simulink model "nonlinear_simulation_stabilization"  (R2023a)
settings: Solver=VariableStepAuto  StartTime=0.0  StopTime=10.0  RelTol=1e-3
model workspace: external: MATLAB File C:\Uni\Projektarbeit\matlab\nonlinear_fo_prep.m (data not in the file)
undefined symbols (not defined in the file): C_out, init_cond
settings Model: Creator=morit  LastModifiedBy=morit

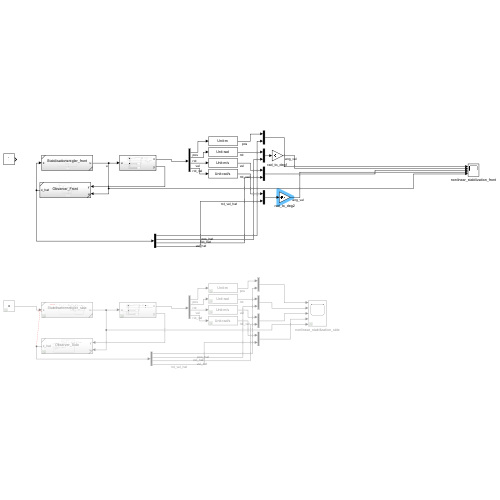
[thumbnail: Simulink's stored preview of the top-level diagram]
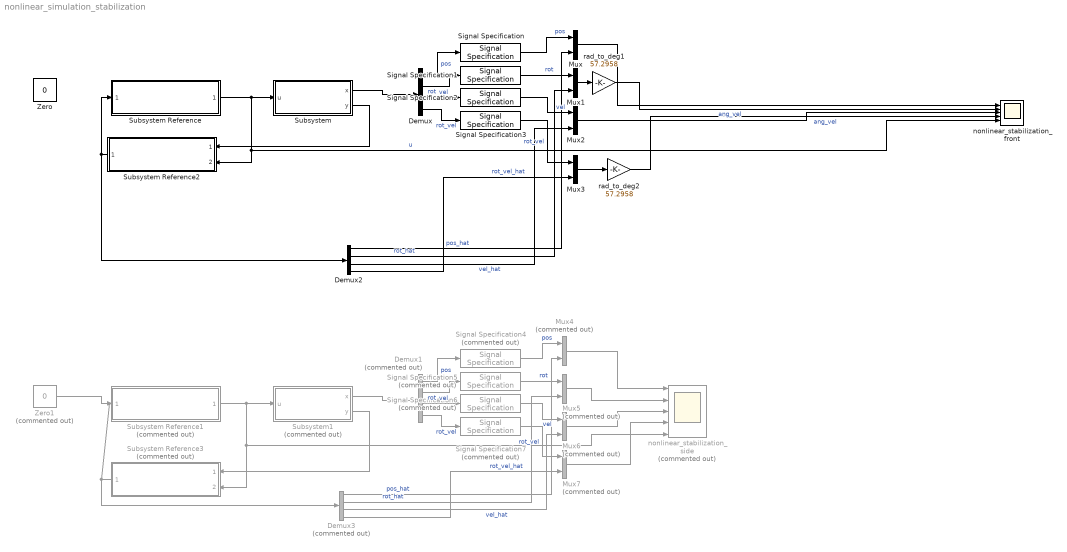
== system nonlinear_simulation_stabilization ==
  Demux : Demux
  Demux1 : Demux  Commented=on
  Demux2 : Demux
  Demux3 : Demux  Commented=on
  Mux{,1..3} (4 alike) : Mux  Inputs=2
  Mux{4..7} (4 alike) : Mux  Commented=on  Inputs=2
  Signal Specification : SignalSpecification  Unit=m
  Signal Specification1 : SignalSpecification  Unit=rad
  Signal Specification2 : SignalSpecification  Unit=m/s
  Signal Specification3 : SignalSpecification  Unit=rad/s
  Signal Specification4 : SignalSpecification  Commented=on  Unit=m
  Signal Specification5 : SignalSpecification  Commented=on  Unit=rad
  Signal Specification6 : SignalSpecification  Commented=on  Unit=m/s
  Signal Specification7 : SignalSpecification  Commented=on  Unit=rad/s
  Subsystem : Subsystem
  Subsystem Reference : Subsystem  ReferencedSubsystem=Stabilisationsregler_front
  Subsystem Reference1 : Subsystem  Commented=on  ReferencedSubsystem=Stabilisationsregler_side
  Subsystem Reference2 : Subsystem  ReferencedSubsystem=Observer_Front
  Subsystem Reference3 : Subsystem  Commented=on  ReferencedSubsystem=Observer_Side
  Subsystem1 : Subsystem  Commented=on
  Zero : Constant  Value=0  OutDataTypeStr=Inherit: Inherit via back propagation
  Zero1 : Constant  Commented=on  Value=0  OutDataTypeStr=Inherit: Inherit via back propagation
  nonlinear_stabilization_front : Scope  NumInputPorts=5
  nonlinear_stabilization_side : Scope  Commented=on  NumInputPorts=5
  rad_to_deg1 : Gain  Gain=57.2958
  rad_to_deg2 : Gain  Gain=57.2958
  wires:
  Subsystem Reference/1 -> Subsystem Reference2/2, nonlinear_stabilization_front/5, Subsystem/1(u)  "u"
  Subsystem/1(x) -> Demux/1
  Demux/3 -> Signal Specification2/1  "vel"
  Demux/1 -> Signal Specification/1  "pos"
  Signal Specification/1 -> Mux/1  "pos"
  Demux/2 -> Signal Specification1/1  "rot"
  Demux/4 -> Signal Specification3/1  "rot_vel"
  Demux1/3 -> Signal Specification6/1  "vel"
  Subsystem1/1(x) -> Demux1/1
  Demux1/1 -> Signal Specification4/1  "pos"
  Subsystem Reference1/1 -> nonlinear_stabilization_side/5, Subsystem Reference3/2, Subsystem1/1(u)
  Demux1/2 -> Signal Specification5/1  "rot"
  Zero1/1 -> Subsystem Reference1/1
  Demux1/4 -> Signal Specification7/1  "rot_vel"
  Subsystem/2(y) -> Subsystem Reference2/1
  Subsystem Reference2/1 -> Demux2/1, Subsystem Reference/1
  Signal Specification1/1 -> Mux1/1  "rot"
  Signal Specification2/1 -> Mux2/1  "vel"
  Signal Specification3/1 -> Mux3/1  "rot_vel"
  Demux2/1 -> Mux/2  "pos_hat"
  Demux2/2 -> Mux1/2  "rot_hat"
  Demux2/3 -> Mux2/2  "vel_hat"
  Demux2/4 -> Mux3/2  "rot_vel_hat"
  Mux/1 -> nonlinear_stabilization_front/1
  Mux1/1 -> rad_to_deg1/1
  Mux2/1 -> nonlinear_stabilization_front/3
  Mux3/1 -> rad_to_deg2/1
  Subsystem1/2(y) -> Subsystem Reference3/1
  Subsystem Reference3/1 -> Demux3/1
  Signal Specification4/1 -> Mux4/1  "pos"
  Signal Specification5/1 -> Mux5/1  "rot"
  Signal Specification6/1 -> Mux6/1  "vel"
  Signal Specification7/1 -> Mux7/1  "rot_vel"
  Demux3/1 -> Mux4/2  "pos_hat"
  Demux3/3 -> Mux6/2  "vel_hat"
  Demux3/2 -> Mux5/2  "rot_hat"
  Demux3/4 -> Mux7/2  "rot_vel_hat"
  Mux4/1 -> nonlinear_stabilization_side/1
  Mux5/1 -> nonlinear_stabilization_side/2
  Mux6/1 -> nonlinear_stabilization_side/3
  Mux7/1 -> nonlinear_stabilization_side/4
  rad_to_deg1/1 -> nonlinear_stabilization_front/2  "ang_vel"
  rad_to_deg2/1 -> nonlinear_stabilization_front/4  "ang_vel"

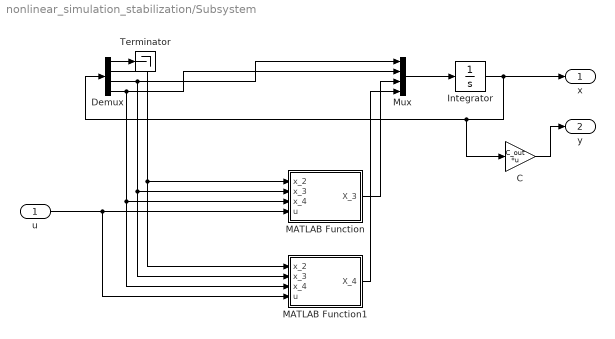
== system nonlinear_simulation_stabilization/Subsystem ==
  u : Inport
  C : Gain  Gain=C_out  Multiplication=Matrix(K*u)
  Demux : Demux
  Integrator : Integrator  InitialCondition=init_cond
  MATLAB Function : MATLAB Function  TreatAsAtomicUnit=on
  MATLAB Function1 : MATLAB Function  TreatAsAtomicUnit=on
  Mux : Mux
  Terminator : Terminator
  x : Outport
  y : Outport  Port=2
  wires:
  u/1 -> MATLAB Function1/4(u), MATLAB Function/4(u)
  Integrator/1 -> C/1, Demux/1, x/1
  Mux/1 -> Integrator/1
  Demux/3 -> MATLAB Function1/2(x_3), MATLAB Function/2(x_3), Mux/1
  Demux/4 -> MATLAB Function1/3(x_4), MATLAB Function/3(x_4), Mux/2
  Demux/2 -> MATLAB Function1/1(x_2), MATLAB Function/1(x_2)
  MATLAB Function/1(X_3) -> Mux/3
  MATLAB Function1/1(X_4) -> Mux/4
  Demux/1 -> Terminator/1
  C/1 -> y/1

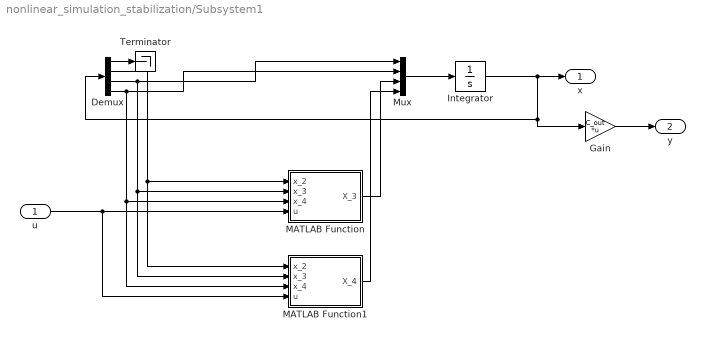
== system nonlinear_simulation_stabilization/Subsystem1 ==
  u : Inport
  Demux : Demux
  Gain : Gain  Gain=C_out  Multiplication=Matrix(K*u)
  Integrator : Integrator  InitialCondition=init_cond
  MATLAB Function : MATLAB Function  TreatAsAtomicUnit=on
  MATLAB Function1 : MATLAB Function  TreatAsAtomicUnit=on
  Mux : Mux
  Terminator : Terminator
  x : Outport
  y : Outport  Port=2
  wires:
  u/1 -> MATLAB Function1/4(u), MATLAB Function/4(u)
  Integrator/1 -> Gain/1, Demux/1, x/1
  Mux/1 -> Integrator/1
  Demux/3 -> MATLAB Function1/2(x_3), MATLAB Function/2(x_3), Mux/1
  Demux/4 -> MATLAB Function1/3(x_4), MATLAB Function/3(x_4), Mux/2
  Demux/2 -> MATLAB Function1/1(x_2), MATLAB Function/1(x_2)
  MATLAB Function/1(X_3) -> Mux/3
  MATLAB Function1/1(X_4) -> Mux/4
  Demux/1 -> Terminator/1
  Gain/1 -> y/1

== matlab function nonlinear_simulation_stabilization/Subsystem/MATLAB Function1 ==
  data: x_2 input; x_3 input; x_4 input; u input; X_4 output
function X_4 = fcn(x_2, x_3, x_4, u)

X_4 = -(33.614*(0.00012941*cos(x_2)*sin(x_2)*x_4^2 + 0.0088444*sin(x_2) + 0.03792*cos(x_2)*(0.48*x_3 - 0.079*u)))/(0.00435*cos(x_2)^2 - 0.004558);

== matlab function nonlinear_simulation_stabilization/Subsystem/MATLAB Function ==
  data: x_2 input; x_3 input; x_4 input; u input; X_3 output
function X_3 = fcn(x_2, x_3, x_4, u)

X_3 = (0.39939*(0.0016381*sin(x_2)*x_4^2 + 0.2304*x_3 - 0.03792*u + 0.10685*cos(x_2)*sin(x_2)))/(0.00435*cos(x_2)^2 - 0.004558);

== matlab function nonlinear_simulation_stabilization/Subsystem1/MATLAB Function ==
  data: x_2 input; x_3 input; x_4 input; u input; X_3 output
function X_3 = fcn(x_2, x_3, x_4, u)

X_3 = (0.25932*(0.00033747*sin(x_2)*x_4^2 + 0.2304*x_3 - 0.012024*u + 0.017424*cos(x_2)*sin(x_2)))/(0.00046059*cos(x_2)^2 - 0.00047314);

== matlab function nonlinear_simulation_stabilization/Subsystem1/MATLAB Function1 ==
  data: x_2 input; x_3 input; x_4 input; u input; X_4 output
function X_4 = fcn(x_2, x_3, x_4, u)

X_4 = -(54.484*(8.4536e-6*cos(x_2)*sin(x_2)*x_4^2 + 0.00044837*sin(x_2) + 0.012024*cos(x_2)*(0.48*x_3 - 0.02505*u)))/(0.00046059*cos(x_2)^2 - 0.00047314);
